simulink model "gm_sampleModel1573_sub_sub"  (R2023a)
settings: Solver=VariableStepAuto  StartTime=0.0  StopTime=10.0  RelTol=1e-3
libraries: simulink x2, hdlsllib x2
settings Model: Creator=user1  LastModifiedBy=user1
settings OptimizationCC: BlockReduction=off  ConditionallyExecuteInputs=off
settings DebuggingCC: InheritedTsInSrcMsg=none

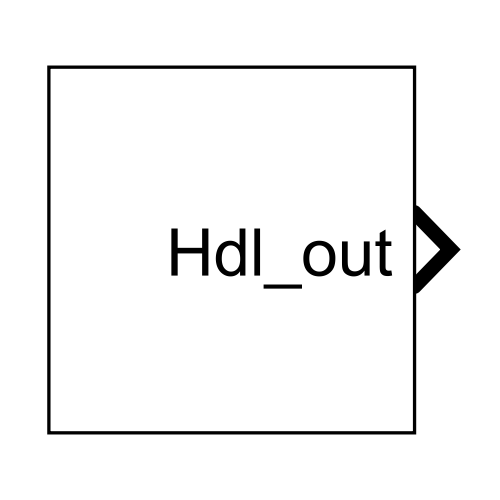
[thumbnail: Simulink's stored preview of the top-level diagram]
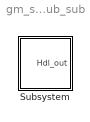
== system gm_sampleModel1573_sub_sub ==
  Subsystem : Subsystem

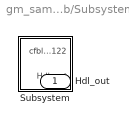
== system gm_sampleModel1573_sub_sub/Subsystem ==
  Subsystem : Subsystem
  Hdl_out : Outport  OutDataTypeStr=uint8

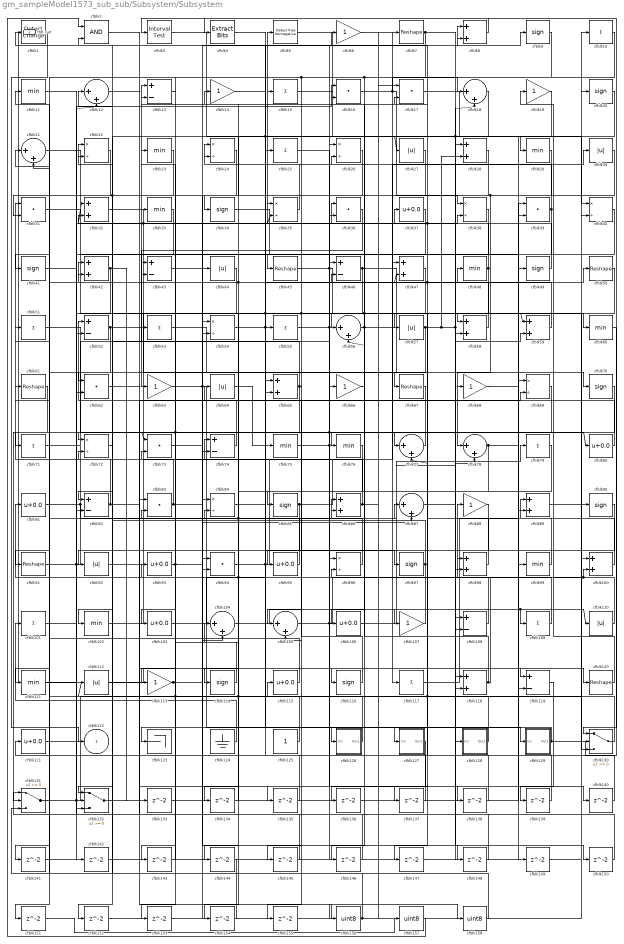
== system gm_sampleModel1573_sub_sub/Subsystem/Subsystem ==
  cfblk1 : simulink/Logic and Bit Operations/Detect Change  vinit=0  OutDataTypeStr=uint8
      settings: LibrarySourceBlock=|
      | hdlsllib/Logic and Bit
      | Operations/Detect
      | Change
  cfblk{10,15,25,51,53,55,71,79,101,109,117} (11 alike) : Sum  Inputs=+  OutDataTypeStr=uint8
  cfblk{8,28,32,42,47,58..59,65,86,89,98,100,118} (13 alike) : Sum  OutDataTypeStr=uint8
  cfblk{11,23,29,33,48,60,75..76,99,102,111} (11 alike) : MinMax  OutDataTypeStr=uint8
  cfblk{37,80..81,93,95,103,106,115,121} (9 alike) : Bias  Bias=0.0  SaturateOnIntegerOverflow=off
  cfblk{12,18,21,56,77..78,87,104..105} (9 alike) : Sum  Inputs=|++  OutDataTypeStr=uint8
  cfblk{6,14,19,63,66,68,88,107,113} (9 alike) : Gain  OutDataTypeStr=uint8
  cfblk{13,43,46,52,74,82,108,119} (8 alike) : Sum  Inputs=+-  OutDataTypeStr=uint8
  cfblk{27,30,44,57,64,92,110,112} (8 alike) : Abs  OutDataTypeStr=uint8  SaturateOnIntegerOverflow=off
  cfblk{9,20,34,41,49,70,85,90,97,114,116} (11 alike) : Signum
  cfblk{7,45,50,61,67,91,120} (7 alike) : Reshape
  cfblk123 : Terminator
  cfblk124 : Ground
  cfblk125 : Constant  OutDataTypeStr=uint8  SampleTime=-1
  cfblk126 : Subsystem
      settings: LibrarySourceBlock=|
      | hdlsllib/Ports &
      | Subsystems/Subsystem
  cfblk127 : Subsystem
      settings: LibrarySourceBlock=|
      | hdlsllib/Ports &
      | Subsystems/Subsystem
  cfblk128 : Subsystem
      settings: LibrarySourceBlock=|
      | hdlsllib/Ports &
      | Subsystems/Subsystem
  cfblk129 : Subsystem
      settings: LibrarySourceBlock=|
      | hdlsllib/Ports &
      | Subsystems/Subsystem
  cfblk130 : Switch  OutDataTypeStr=uint8  SaturateOnIntegerOverflow=off  InputSameDT=off
  cfblk131 : Switch  OutDataTypeStr=uint8  SaturateOnIntegerOverflow=off  InputSameDT=off
  cfblk132 : Switch  OutDataTypeStr=uint8  SaturateOnIntegerOverflow=off  InputSameDT=off
  cfblk{133..155} (23 alike) : Delay  SampleTime=1
  cfblk156 : DataTypeConversion  OutDataTypeStr=uint8  SaturateOnIntegerOverflow=off  RndMeth=Floor
  cfblk157 : DataTypeConversion  OutDataTypeStr=uint8  SaturateOnIntegerOverflow=off  RndMeth=Floor
  cfblk158 : DataTypeConversion  OutDataTypeStr=uint8  SaturateOnIntegerOverflow=off  RndMeth=Floor
  cfblk{16..17,31,36,39,62,73,83,94} (9 alike) : DotProduct  OutDataTypeStr=uint8
  cfblk2 : Logic  AllPortsSameDT=off  OutDataTypeStr=boolean
  cfblk{22,24,26,35,38,40,54,69,72,84,96} (11 alike) : Product  Inputs=*/  OutDataTypeStr=uint8  RndMeth=Zero  SaturateOnIntegerOverflow=on
  cfblk3 : hdlsllib/Logic and Bit Operations/Interval Test  IntervalClosedRight=on  uplimit=0.5  IntervalClosedLeft=on  lowlimit=-0.5  OutDataTypeStr=uint8
  cfblk4 : simulink/Logic and Bit Operations/Extract Bits  bitsToExtract=Upper half  numBits=8  bitIdxRange=[0 7]  outScalingMode=Preserve fixed-point scaling
      settings: LibrarySourceBlock=|
      | hdlsllib/Logic and Bit
      | Operations/Extract Bits
  cfblk5 : hdlsllib/Logic and Bit Operations/Detect Rise Nonnegative  vinit=0  OutDataTypeStr=uint8
  cfblk122 : Outport  OutDataTypeStr=uint8  VectorParamsAs1DForOutWhenUnconnected=off
  Hdl_out : Outport  Port=2  OutDataTypeStr=uint8
  wires:
  cfblk109/1 -> cfblk88/1
  cfblk126/1(Out1) -> cfblk93/1, cfblk112/1
  cfblk124/1 -> cfblk101/1
  cfblk86/1 -> cfblk32/2, cfblk7/1
  cfblk38/1 -> cfblk45/1
  cfblk53/1 -> cfblk67/1
  cfblk83/1 -> cfblk87/2, cfblk56/1
  cfblk92/1 -> cfblk79/1
  cfblk55/1 -> cfblk8/1, cfblk118/2, cfblk80/1
  cfblk64/1 -> cfblk75/1
  cfblk70/1 -> cfblk77/1
  cfblk46/1 -> cfblk144/1, cfblk70/1
  cfblk40/1 -> cfblk58/1
  cfblk36/1 -> cfblk63/1
  cfblk84/1 -> cfblk46/2, cfblk55/1
  cfblk16/1 -> cfblk60/1, cfblk18/1, cfblk38/1
  cfblk82/1 -> cfblk69/2, cfblk31/1
  cfblk130/1 -> cfblk83/2, cfblk77/2
  cfblk49/1 -> cfblk5/1
  cfblk35/1 -> cfblk15/1
  cfblk128/1(Out1) -> cfblk51/1
  cfblk78/1 -> cfblk147/1, cfblk49/1
  cfblk61/1 -> cfblk71/1
  cfblk39/1 -> cfblk82/2, cfblk24/1
  cfblk54/1 -> cfblk9/1, cfblk59/1
  cfblk62/1 -> cfblk120/1
  cfblk63/1 -> cfblk148/1, cfblk129/1(In1)
  cfblk74/1 -> cfblk52/1
  cfblk71/1 -> cfblk13/1
  cfblk56/1 -> cfblk106/1, cfblk99/1
  cfblk32/1 -> cfblk35/2, cfblk78/1
  cfblk47/1 -> cfblk146/1, cfblk145/1
  cfblk106/1 -> cfblk28/1
  cfblk21/1 -> cfblk117/1
  cfblk28/1 -> cfblk94/2
  cfblk66/1 -> cfblk36/1
  cfblk24/1 -> cfblk41/1
  cfblk120/1 -> cfblk89/1
  cfblk51/1 -> cfblk78/2
  cfblk20/1 -> cfblk108/2, cfblk34/1
  cfblk103/1 -> cfblk65/2
  cfblk94/1 -> cfblk87/1, cfblk30/1
  cfblk17/1 -> cfblk40/1
  cfblk129/1(Out1) -> cfblk123/1, cfblk3/1
  cfblk37/1 -> cfblk113/1, cfblk73/1
  cfblk15/1 -> cfblk29/1
  cfblk80/1 -> cfblk42/1
  cfblk50/1 -> cfblk155/1, cfblk54/2
  cfblk108/1 -> cfblk81/1
  cfblk93/1 -> cfblk153/1, cfblk86/1
  cfblk34/1 -> cfblk66/1
  cfblk41/1 -> cfblk37/1
  cfblk121/1 -> cfblk115/1
  cfblk77/1 -> cfblk76/1
  cfblk97/1 -> cfblk96/2, cfblk42/2
  cfblk131/1 -> cfblk12/2, cfblk20/1
  cfblk42/1 -> cfblk133/1, cfblk62/2
  cfblk112/1 -> cfblk116/1
  cfblk60/1 -> cfblk130/1
  cfblk96/1 -> cfblk11/1
  cfblk115/1 -> cfblk61/1
  cfblk81/1 -> cfblk86/2, cfblk46/1
  cfblk116/1 -> cfblk64/1
  cfblk91/1 -> cfblk16/1, cfblk25/1
  cfblk1/1 -> cfblk122/1
  cfblk102/1 -> cfblk50/1
  cfblk117/1 -> cfblk39/1
  cfblk75/1 -> cfblk48/1, cfblk110/1, cfblk109/1
  cfblk110/1 -> cfblk100/2, cfblk19/1
  cfblk6/1 -> cfblk119/1
  cfblk73/1 -> cfblk104/2
  cfblk7/1 -> cfblk105/2, cfblk128/1(In1)
  cfblk26/1 -> cfblk132/1
  cfblk98/1 -> cfblk13/2
  cfblk3/1 -> cfblk108/1
  cfblk19/1 -> cfblk119/2
  cfblk2/1 -> cfblk156/1
  cfblk31/1 -> cfblk69/1
  cfblk14/1 -> cfblk27/1, cfblk126/1(In1)
  cfblk111/1 -> cfblk52/2
  cfblk57/1 -> cfblk151/1, cfblk28/2, cfblk18/2, cfblk59/2
  cfblk27/1 -> cfblk36/2
  cfblk22/1 -> cfblk111/1
  cfblk5/1 -> cfblk47/1
  cfblk114/1 -> cfblk23/1
  cfblk118/1 -> cfblk16/2, cfblk98/1
  cfblk58/1 -> cfblk24/2, cfblk21/1
  cfblk79/1 -> cfblk114/1
  cfblk52/1 -> cfblk132/3, cfblk89/2
  cfblk72/1 -> cfblk12/1
  cfblk69/1 -> cfblk143/1, cfblk131/2
  cfblk99/1 -> cfblk1/1
  cfblk113/1 -> Hdl_out/1, cfblk6/1
  cfblk100/1 -> cfblk47/2, cfblk32/1, cfblk26/2
  cfblk44/1 -> cfblk92/1
  cfblk89/1 -> cfblk90/1
  cfblk88/1 -> cfblk127/1(In1)
  cfblk8/1 -> cfblk4/1
  cfblk23/1 -> cfblk91/1
  cfblk45/1 -> cfblk57/1, cfblk130/3
  cfblk33/1 -> cfblk72/1
  cfblk29/1 -> cfblk62/1
  cfblk48/1 -> cfblk137/1, cfblk33/1
  cfblk104/1 -> cfblk107/1
  cfblk9/1 -> cfblk56/2, cfblk53/1, cfblk95/1
  cfblk4/1 -> cfblk97/1
  cfblk107/1 -> cfblk43/2, cfblk84/2
  cfblk85/1 -> cfblk38/2, cfblk102/1
  cfblk13/1 -> cfblk103/1
  cfblk30/1 -> cfblk68/1, cfblk82/1, cfblk31/2
  cfblk125/1 -> cfblk72/2, cfblk74/1
  cfblk132/1 -> cfblk44/1
  cfblk76/1 -> cfblk105/1
  cfblk105/1 -> cfblk8/2, cfblk10/1
  cfblk59/1 -> cfblk43/1
  cfblk65/1 -> cfblk74/2, cfblk22/1, cfblk85/1
  cfblk95/1 -> cfblk22/2, cfblk14/1
  cfblk101/1 -> cfblk35/1
  cfblk133/1 -> cfblk58/2
  cfblk90/1 -> cfblk134/1
  cfblk134/1 -> cfblk104/1
  cfblk43/1 -> cfblk135/1
  cfblk135/1 -> cfblk65/1
  cfblk127/1(Out1) -> cfblk136/1
  cfblk136/1 -> cfblk39/2
  cfblk137/1 -> cfblk21/2
  cfblk12/1 -> cfblk138/1
  cfblk138/1 -> cfblk17/2
  cfblk119/1 -> cfblk139/1
  cfblk139/1 -> cfblk118/1
  cfblk25/1 -> cfblk140/1
  cfblk140/1 -> cfblk26/1
  cfblk10/1 -> cfblk141/1
  cfblk141/1 -> cfblk100/1
  cfblk11/1 -> cfblk142/1
  cfblk142/1 -> cfblk96/1
  cfblk143/1 -> cfblk73/2
  cfblk144/1 -> cfblk131/3
  cfblk145/1 -> cfblk94/1
  cfblk146/1 -> cfblk131/1
  cfblk147/1 -> cfblk98/2
  cfblk148/1 -> cfblk132/2
  cfblk68/1 -> cfblk149/1
  cfblk149/1 -> cfblk130/2
  cfblk87/1 -> cfblk150/1
  cfblk150/1 -> cfblk83/1
  cfblk18/1 -> cfblk152/1
  cfblk152/1 -> cfblk84/1
  cfblk153/1 -> cfblk40/2
  cfblk67/1 -> cfblk154/1
  cfblk154/1 -> cfblk54/1
  cfblk156/1 -> cfblk17/1, cfblk121/1
  cfblk151/1 -> cfblk157/1
  cfblk157/1 -> cfblk2/1
  cfblk155/1 -> cfblk158/1
  cfblk158/1 -> cfblk2/2

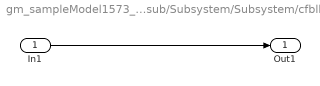
== system gm_sampleModel1573_sub_sub/Subsystem/Subsystem/cfblk126 ==
  In1 : Inport
  Out1 : Outport
  wires:
  In1/1 -> Out1/1

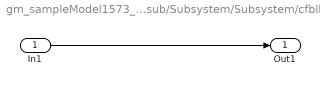
== system gm_sampleModel1573_sub_sub/Subsystem/Subsystem/cfblk127 ==
  In1 : Inport
  Out1 : Outport
  wires:
  In1/1 -> Out1/1

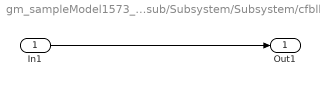
== system gm_sampleModel1573_sub_sub/Subsystem/Subsystem/cfblk128 ==
  In1 : Inport
  Out1 : Outport
  wires:
  In1/1 -> Out1/1

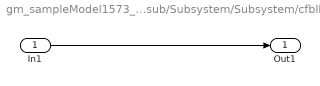
== system gm_sampleModel1573_sub_sub/Subsystem/Subsystem/cfblk129 ==
  In1 : Inport
  Out1 : Outport
  wires:
  In1/1 -> Out1/1
